simulink model "timegaptest"  (R2023b)
settings: Solver=ode4  StartTime=0.0  StopTime=10.0  FixedStep=0.001  RelTol=1e-3
values from neighbouring files (symbols this model uses):
  B = 0.0003    [Scenario 1, 2.mat]    (also in motor_parameter_gw.m; motor_parameter_gw_v2.m; sampleScenario_gw_v0.1.mat)
  J = 2.09e-05    [Scenario 1, 2.mat]    (also in motor_parameter_gw.m; motor_parameter_gw_v2.m; sampleScenario_gw_v0.1.mat)
  Kb = 0.042    [Scenario 1, 2.mat]    (also in motor_parameter_gw.m; motor_parameter_gw_v2.m; sampleScenario_gw_v0.1.mat)
  Kdi = 0.5    [Scenario 1, 2.mat]    (also in motor_parameter_gw.m; motor_parameter_gw_v2.m = 3.9; sampleScenario_gw_v0.1.mat)
  Kdp = 1    [Scenario 1, 2.mat]    (also in motor_parameter_gw.m; motor_parameter_gw_v2.m = 4; sampleScenario_gw_v0.1.mat)
  Ki = 0.8    [Scenario 1, 2.mat]    (also in motor_parameter_gw.m; motor_parameter_gw_v2.m = 0.9; sampleScenario_gw_v0.1.mat)
  Kp = 0.5    [Scenario 1, 2.mat]    (also in motor_parameter_gw.m; motor_parameter_gw_v2.m = 0.3; sampleScenario_gw_v0.1.mat)
  Kt = 0.042    [Scenario 1, 2.mat]    (also in motor_parameter_gw.m; motor_parameter_gw_v2.m; sampleScenario_gw_v0.1.mat)
  L = 1.16    [Scenario 1, 2.mat]    (also in motor_parameter_gw.m; motor_parameter_gw_v2.m; sampleScenario_gw_v0.1.mat)
  Ldes = 20    [Scenario 1, 2.mat]    (also in motor_parameter_gw.m; motor_parameter_gw_v2.m; sampleScenario_gw_v0.1.mat)
  R = 8.4    [Scenario 1, 2.mat]    (also in motor_parameter_gw.m; motor_parameter_gw_v2.m; sampleScenario_gw_v0.1.mat)
  Wconst = 60    [Scenario 1, 2.mat]    (also in motor_parameter_gw.m; motor_parameter_gw_v2.m; sampleScenario_gw_v0.1.mat)
libraries: SignalEditorBlockLib x1, arduinosensorlib x1
settings Model: Creator=현대오토1  LastModifiedBy=현대오토1

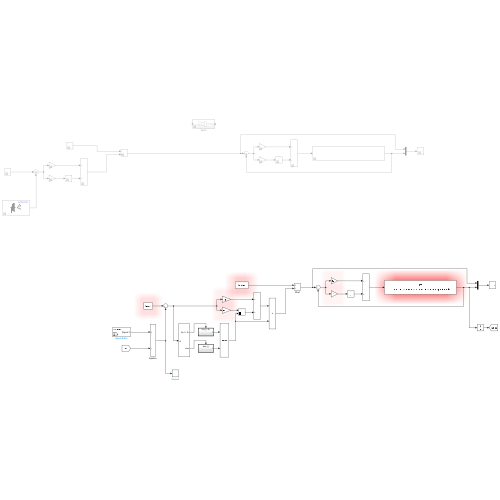
[thumbnail: Simulink's stored preview of the top-level diagram]
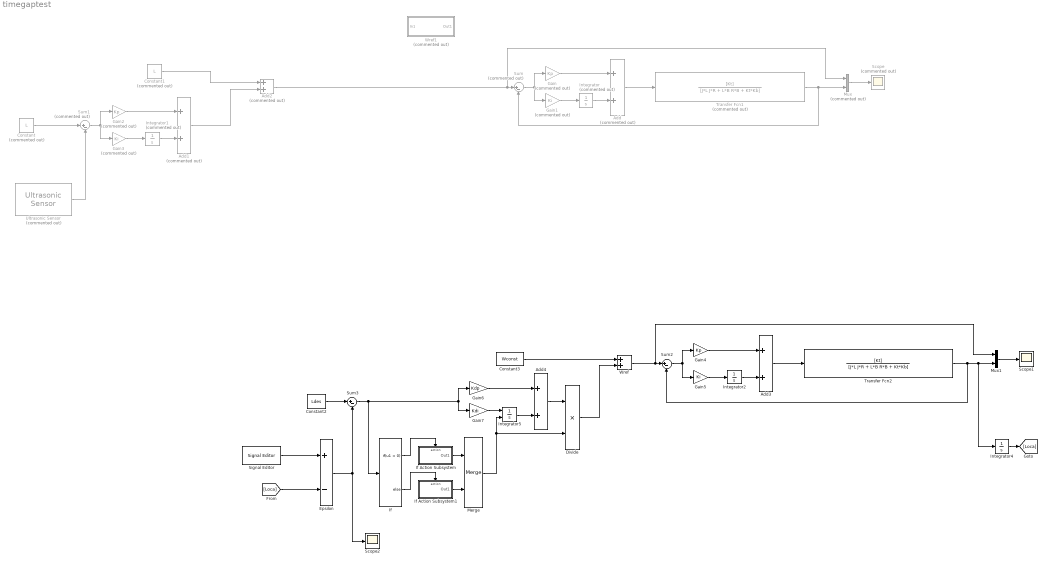
== system timegaptest ==
  Add : Sum  Commented=on
  Add1 : Sum  Commented=on
  Add2 : Sum  Commented=on
  Add3 : Sum
  Add4 : Sum
  Constant : Constant  Commented=on  Value=L
  Constant1 : Constant  Commented=on  Value=L
  Constant2 : Constant  Value=Ldes
  Constant3 : Constant  Value=Wconst
  Divide : Product
  Epsilon : Sum  Inputs=+-
  Gain : Gain  Commented=on  Gain=Kp
  Gain1 : Gain  Commented=on  Gain=Ki
  Gain2 : Gain  Commented=on  Gain=Kp
  Gain3 : Gain  Commented=on  Gain=Ki
  Gain4 : Gain  Gain=Kp
  Gain5 : Gain  Gain=Ki
  Gain6 : Gain  Gain=Kdp
  Gain7 : Gain  Gain=Kdi
  If : If  IfExpression=u1 < 0
  If Action Subsystem : Subsystem  TreatAsAtomicUnit=on
  If Action Subsystem1 : Subsystem  TreatAsAtomicUnit=on
  Integrator : Integrator  Commented=on
  Integrator1 : Integrator  Commented=on
  Integrator2 : Integrator
  Integrator4 : Integrator  InitialCondition=3
  Integrator5 : Integrator  ExternalReset=either
  Merge : Merge
  Mux : Mux  Commented=on  Inputs=2
  Mux1 : Mux  Inputs=2
  Scope : Scope  Commented=on
  Scope1 : Scope
  Scope2 : Scope
  Signal Editor : SignalEditorBlockLib/Signal Editor  FileName=untitled.mat  ActiveScenario=Scenario  ActiveSignal=Signal 1  IsBus=off  OutputBusObjectStr=Bus: BusObject  SampleTime=0  Interpolate=off  ZeroCross=off  OutputAfterFinalValue=Setting to zero  Unit=inherit  PreserveSignalName=on  ApplySigPropsToAllScenarios=on  ApplySigPropsToAllSignals=off
  Sum : Sum  Commented=on  Inputs=|+-
  Sum1 : Sum  Commented=on  Inputs=|+-
  Sum2 : Sum  Inputs=|+-
  Sum3 : Sum  Inputs=|+-
  Transfer Fcn1 : TransferFcn  Commented=on  Numerator=[Kt]  Denominator=[J*L J*R + L*B R*B + Kt*Kb]
  Transfer Fcn2 : TransferFcn  Numerator=[Kt]  Denominator=[J*L J*R + L*B R*B + Kt*Kb]
  Ultrasonic Sensor : arduinosensorlib/Ultrasonic Sensor  Commented=on  NumSignalPins=1  TrigPin=4  EchoPin=5  SignalPin=3  SampleTime_=0.1  blockPlatform=ARDUINO
  Wref : Sum
  Wref1 : Subsystem  Commented=on
  wires:
  Sum/1 -> Gain/1, Gain1/1
  Gain1/1 -> Integrator/1
  Gain/1 -> Add/1
  Integrator/1 -> Add/2
  Add/1 -> Transfer Fcn1/1
  Add2/1 -> Mux/1, Sum/1
  Transfer Fcn1/1 -> Mux/2, Sum/2
  Mux/1 -> Scope/1
  Constant/1 -> Sum1/1
  Gain3/1 -> Integrator1/1
  Integrator1/1 -> Add1/2
  Sum1/1 -> Gain2/1, Gain3/1
  Gain2/1 -> Add1/1
  Add1/1 -> Add2/2
  Ultrasonic Sensor/1 -> Sum1/2
  Constant1/1 -> Add2/1
  Constant3/1 -> Wref/1
  Constant2/1 -> Sum3/1
  Gain5/1 -> Integrator2/1
  Gain6/1 -> Add4/1
  Sum3/1 -> If/1, Gain6/1, Gain7/1
  Gain7/1 -> Integrator5/1
  Integrator5/1 -> Add4/2
  Integrator2/1 -> Add3/2
  Wref/1 -> Mux1/1, Sum2/1
  Sum2/1 -> Gain4/1, Gain5/1
  Gain4/1 -> Add3/1
  Transfer Fcn2/1 -> Integrator4/1, Mux1/2, Sum2/2
  Add3/1 -> Transfer Fcn2/1
  Mux1/1 -> Scope1/1
  Integrator4/1 -> [Loca]
  [Loca] -> Epsilon/2
  Signal Editor/1 -> Epsilon/1
  Epsilon/1 -> Scope2/1, Sum3/2
  If/1 -> If Action Subsystem/Action
  If/2 -> If Action Subsystem1/Action
  If Action Subsystem/1(Out1) -> Merge/1
  If Action Subsystem1/1(Out1) -> Merge/2
  Merge/1 -> Divide/2, Integrator5/2
  Add4/1 -> Divide/1
  Divide/1 -> Wref/2

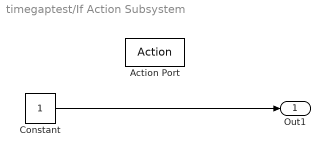
== system timegaptest/If Action Subsystem ==
  Action Port : ActionPort  ActionPortLabel=if(u1 < 0)
  Constant : Constant
  Out1 : Outport
  wires:
  Constant/1 -> Out1/1

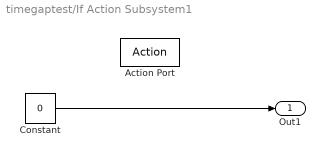
== system timegaptest/If Action Subsystem1 ==
  Action Port : ActionPort  ActionPortLabel=else
  Constant : Constant  Value=0
  Out1 : Outport
  wires:
  Constant/1 -> Out1/1

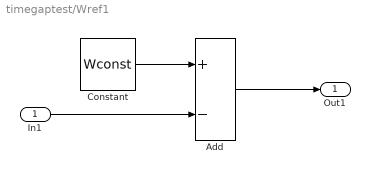
== system timegaptest/Wref1 ==
  In1 : Inport
  Add : Sum  Inputs=+-
  Constant : Constant  Value=Wconst
  Out1 : Outport
  wires:
  Add/1 -> Out1/1
  In1/1 -> Add/2
  Constant/1 -> Add/1
